simulink model "Parte1_SeccionC_Sistemareal"  (R2021a)
settings: Solver=VariableStepAuto  StartTime=0.0  StopTime=10000.0  RelTol=1e-3
values from neighbouring files (symbols this model uses):
  A = 3    [Tarea1Parte1SeccionE.m]    (also in Tarea1_Parte1_Todaslassecciones.m; simulink.m)
  g = 9.81    [Tarea1Parte1SeccionE.m]    (also in Tarea1_Parte1_Todaslassecciones.m; Tarea1parte1SeccionD.m; simulink.m)
  Kvs = 0.001    [Tarea1_Parte1_Todaslassecciones.m]    (also in Tarea1parte1SeccionD.m; simulink.m)
  rho = 789    [Tarea1Parte1SeccionE.m]    (also in Tarea1_Parte1_Todaslassecciones.m; Tarea1parte1SeccionD.m; simulink.m)
settings Model: Creator=mluser  LastModifiedBy=mluser

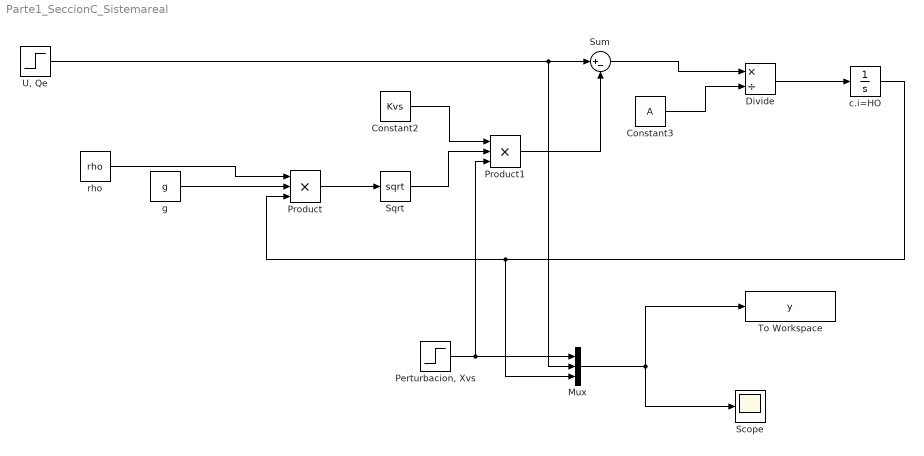
== system Parte1_SeccionC_Sistemareal ==
  Constant2 : Constant  Value=Kvs
  Constant3 : Constant  Value=A
  Divide : Product  Inputs=*/
  Mux : Mux  Inputs=3
  "Perturbacion, Xvs" : Step  Before=1  SampleTime=0
  Product : Product  Inputs=3
  Product1 : Product  Inputs=3
  Scope : Scope
  Sqrt : Sqrt  SaturateOnIntegerOverflow=on
  Sum : Sum  Inputs=|+-
  To Workspace : ToWorkspace  VariableName=y  SaveFormat=Timeseries  SampleTime=-1
  "U, Qe" : Step  Time=2  Before=1  SampleTime=0
  c.i=HO : Integrator
  g : Constant  Value=g
  rho : Constant  Value=rho
  wires:
  "U, Qe"/1 -> Sum/1, Mux/2
  Product1/1 -> Sum/2
  Constant2/1 -> Product1/1
  Product/1 -> Sqrt/1
  Sqrt/1 -> Product1/2
  g/1 -> Product/2
  rho/1 -> Product/1
  c.i=HO/1 -> Product/3, Mux/3
  Sum/1 -> Divide/1
  Constant3/1 -> Divide/2
  Divide/1 -> c.i=HO/1
  Mux/1 -> To Workspace/1, Scope/1
  "Perturbacion, Xvs"/1 -> Mux/1, Product1/3
